simulink library "sensor_processing"  (R2016b)
settings: Solver=VariableStepAuto  StartTime=0.0  StopTime=10.0  RelTol=1e-3
undefined symbols (not defined in the file or in its folder): gyro_omega_body_radps, mag_vec_body_T, sun_vec_body_sunsensor
libraries: MSP_SP x1, bus_stubs_fsw x1
settings Model: Creator=taylorreynolds  LastModifiedBy=Taylor

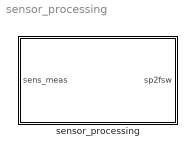
== system sensor_processing ==
  sensor_processing : Subsystem

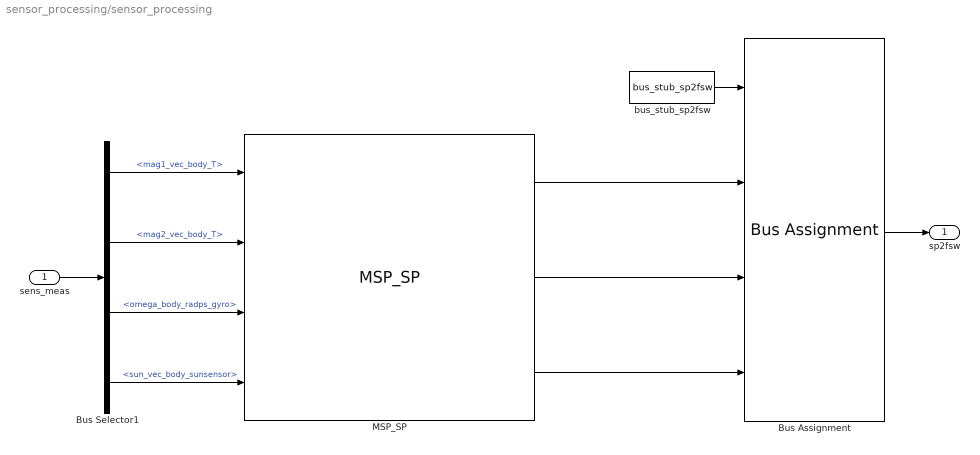
== system sensor_processing/sensor_processing ==
  sens_meas : Inport
  Bus Assignment : BusAssignment  AssignedSignals=mag_vec_body_T,gyro_omega_body_radps,sun_vec_body_sunsensor
  Bus Selector1 : BusSelector  OutputSignals=mag1_vec_body_T,mag2_vec_body_T,omega_body_radps_gyro,sun_vec_body_sunsensor
  MSP_SP : MSP_SP/MSP_SP
  bus_stub_sp2fsw : bus_stubs_fsw/bus_stub_sp2fsw
  sp2fsw : Outport  OutDataTypeStr=Bus: sp2fsw
  wires:
  MSP_SP/2 -> Bus Assignment/3
  Bus Selector1/2 -> MSP_SP/2  "<mag2_vec_body_T>"
  Bus Assignment/1 -> sp2fsw/1
  bus_stub_sp2fsw/1 -> Bus Assignment/1
  sens_meas/1 -> Bus Selector1/1
  Bus Selector1/3 -> MSP_SP/3  "<omega_body_radps_gyro>"
  Bus Selector1/1 -> MSP_SP/1  "<mag1_vec_body_T>"
  Bus Selector1/4 -> MSP_SP/4  "<sun_vec_body_sunsensor>"
  MSP_SP/3 -> Bus Assignment/4
  MSP_SP/1 -> Bus Assignment/2
